simulink model "validation_gate_current"  (Simulink 7.6)
settings: Solver=FixedStepDiscrete  StartTime=0.0  StopTime=0  RelTol=1e-3
values from neighbouring files (symbols this model uses):
  Forward_Camera_Dimensions = [160 120]    [VisionConstants.m]
  Iter_Segment_Thresh = 60    [VisionConstants.m]
undefined symbols (not defined in the file or in its folder): Rec, SDTV
libraries: vipgeotforms x3, vipconversions x2, viptextngfix x1, vipanalysis x1, viptransforms x1
settings Model: Creator=Thing 1  LastModifiedBy=auvt
settings OptimizationCC: OptimizeModelRefInitCode=on
settings RTWCC: SystemTargetFile=ert.tlc  GenCodeOnly=on  TemplateMakefile=ert_default_tmf  Description=Real-Time Workshop Embedded Coder  GenerateReport=on  ProcessScript=ert_make_rtw_hook  IncludeHyperlinkInReport=on  LaunchReport=on  TargetLang=C++
settings CodeAppCC: IgnoreCustomStorageClasses=off
settings ERTTargetCC: MultiwordLength=2048  GenerateSampleERTMain=on  IncludeMdlTerminateFcn=off  ERTCustomFileTemplate=example_file_process.tlc  ConvertIfToSwitch=off

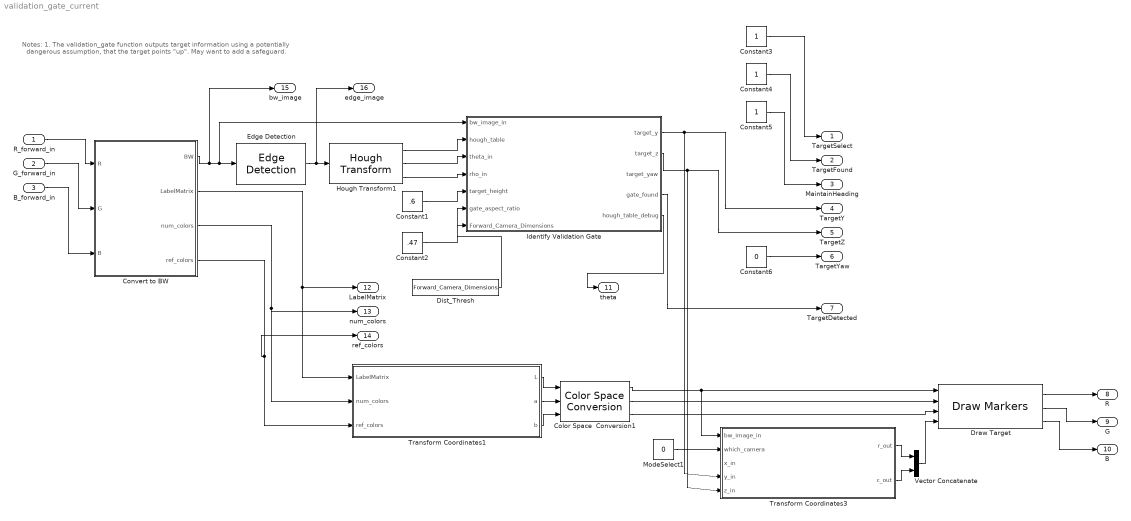
== system validation_gate_current ==
  note: Notes:
      | 1. The validation_gate function outputs target
      | information using a potentially dangerous
      | assumption, that the target points "up". May
      | want to add a safeguard.
  R_forward_in : Inport  PortDimensions=Forward_Camera_Dimensions
  G_forward_in : Inport  Port=2  PortDimensions=Forward_Camera_Dimensions
  B_forward_in : Inport  Port=3  PortDimensions=Forward_Camera_Dimensions
  Color Space  Conversion1 : vipconversions/Color Space  Conversion  conversion=Obsolete  conversionActive=L*a*b* to sR'G'B'  wp_str=D50  rec=Rec. 601 (SDTV)  sys=1125/60/2:1  imagePorts=Separate color signals
  Constant1 : Constant  Value=.6  SampleTime=-1
  Constant2 : Constant  Value=.47  SampleTime=-1
  Constant3 : Constant  SampleTime=-1
  Constant4 : Constant  SampleTime=-1
  Constant5 : Constant  SampleTime=-1
  Constant6 : Constant  Value=0  SampleTime=-1
  Convert to BW : Subsystem
  Dist_Thresh : Constant  Value=Forward_Camera_Dimensions  SampleTime=-1
  Draw Target : viptextngfix/Draw Markers  DialogController=vipDDGCreate  DialogControllerArgs=DataTag3  shape=X-mark  size=7  fill=off  fillClrSource=Specify via dialog  display=User-specified value  intensity=200  color=[0 0 0]  opacity=0.6  viewport=Entire image  antialiasing=off  inType=Obsolete  imagePorts=Separate color signals  prodOutputMode=Binary point scaling  prodOutputWordLength=32  prodOutputFracLength=14  memoryMode=Specify word length  memoryWordLength=16  memoryFracLength=15  roundingMode=Floor  overflowMode=off
  Edge Detection : vipanalysis/Edge Detection  DialogController=vipDDGCreate  DialogControllerArgs=DataTag4  method=Sobel  outputType=Binary image  userDefinedThreshold=off  thresholdSource=Specify via dialog  threshold=20  thresholdTuning=3  edgeThinning=on  threshold_canny=[0.25 0.60]  autoPercent=70  sigma=1  roundingMode=Floor  overflowMode=off
  Hough Transform1 : viptransforms/Hough Transform  DialogController=vipDDGCreate  DialogControllerArgs=DataTag5  theta_res=pi/180  rho_res=1  out_theta_rho=on  outdtmode=double  firstCoeffMode=Binary point scaling  firstCoeffWordLength=16  firstCoeffFracLength=14  secondCoeffMode=Binary point scaling  secondCoeffWordLength=32  secondCoeffFracLength=16  outputMode=Binary point scaling  outputWordLength=16  outputFracLength=0  accumMode=Binary point scaling  accumWordLength=32  accumFracLength=20  prodOutputMode=Binary point scaling  prodOutputWordLength=32  prodOutputFracLength=20  memoryMode=Binary point scaling  memoryWordLength=32  memoryFracLength=16  roundingMode=Nearest  overflowMode=on
  Identify Validation Gate : Stateflow chart  TreatAsAtomicUnit=on  SystemSampleTime=[1/30 0]
  ModeSelect1 : Constant  Value=0  SampleTime=-1
  Transform Coordinates1 : Stateflow chart  TreatAsAtomicUnit=on  SystemSampleTime=[1/30 0]
  Transform Coordinates3 : Stateflow chart  TreatAsAtomicUnit=on  SystemSampleTime=[1/30 0]
  Vector Concatenate : Concatenate  Mode=Multidimensional array
  TargetSelect : Outport  OutDataTypeStr=double
  TargetFound : Outport  Port=2  OutDataTypeStr=double
  MaintainHeading : Outport  Port=3  OutDataTypeStr=double
  TargetY : Outport  Port=4  OutDataTypeStr=double
  TargetZ : Outport  Port=5  OutDataTypeStr=double
  TargetYaw : Outport  Port=6  OutDataTypeStr=double
  TargetDetected : Outport  Port=7  OutDataTypeStr=double
  R : Outport  Port=8  OutDataTypeStr=double
  G : Outport  Port=9  OutDataTypeStr=double
  B : Outport  Port=10  OutDataTypeStr=double
  theta : Outport  Port=11  OutDataTypeStr=double
  LabelMatrix : Outport  Port=12
  num_colors : Outport  Port=13
  ref_colors : Outport  Port=14
  bw_image : Outport  Port=15
  edge_image : Outport  Port=16
  wires:
  Hough Transform1/1 -> Identify Validation Gate/2(hough_table)
  Hough Transform1/2 -> Identify Validation Gate/3(theta_in)
  Hough Transform1/3 -> Identify Validation Gate/4(rho_in)
  Edge Detection/1 -> Hough Transform1/1, edge_image/1
  Constant1/1 -> Identify Validation Gate/5(target_height)
  Constant2/1 -> Identify Validation Gate/6(gate_aspect_ratio)
  Convert to BW/1(BW) -> Edge Detection/1, Identify Validation Gate/1(bw_image_in), bw_image/1
  R_forward_in/1 -> Convert to BW/1(R)
  G_forward_in/1 -> Convert to BW/2(G)
  B_forward_in/1 -> Convert to BW/3(B)
  Identify Validation Gate/1(target_y) -> TargetY/1, Transform Coordinates3/4(y_in)
  Identify Validation Gate/2(target_z) -> TargetZ/1, Transform Coordinates3/5(z_in)
  Identify Validation Gate/4(gate_found) -> TargetDetected/1
  Constant3/1 -> TargetSelect/1
  Constant4/1 -> TargetFound/1
  Constant5/1 -> MaintainHeading/1
  Constant6/1 -> TargetYaw/1
  Vector Concatenate/1 -> Draw Target/4
  Transform Coordinates3/1(r_out) -> Vector Concatenate/1
  Transform Coordinates3/2(c_out) -> Vector Concatenate/2
  ModeSelect1/1 -> Transform Coordinates3/2(which_camera)
  Draw Target/1 -> R/1
  Draw Target/2 -> G/1
  Draw Target/3 -> B/1
  Transform Coordinates1/1(L) -> Color Space  Conversion1/1
  Transform Coordinates1/2(a) -> Color Space  Conversion1/2
  Transform Coordinates1/3(b) -> Color Space  Conversion1/3
  Color Space  Conversion1/1 -> Draw Target/1, Transform Coordinates3/1(bw_image_in)
  Color Space  Conversion1/2 -> Draw Target/2
  Color Space  Conversion1/3 -> Draw Target/3
  Convert to BW/2(LabelMatrix) -> Transform Coordinates1/1(LabelMatrix), LabelMatrix/1
  Convert to BW/3(num_colors) -> Transform Coordinates1/2(num_colors), num_colors/1
  Convert to BW/4(ref_colors) -> Transform Coordinates1/3(ref_colors), ref_colors/1
  Identify Validation Gate/5(hough_table_debug) -> theta/1
  Dist_Thresh/1 -> Identify Validation Gate/7(Forward_Camera_Dimensions)

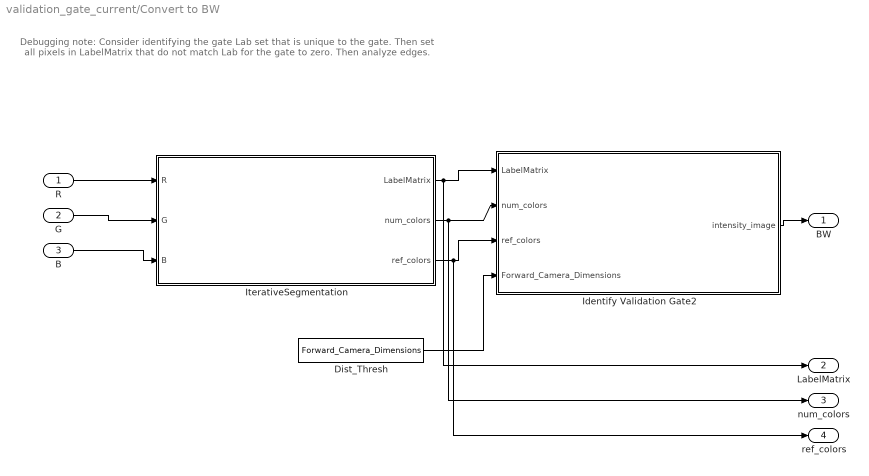
== system validation_gate_current/Convert to BW ==
  note: Debugging note: Consider identifying the gate Lab set that is unique to the gate.
      | Then set all pixels in LabelMatrix that do not match Lab for the gate to zero.
      | Then analyze edges.
  R : Inport  OutDataTypeStr=double
  G : Inport  Port=2  OutDataTypeStr=double
  B : Inport  Port=3  OutDataTypeStr=double
  Dist_Thresh : Constant  Value=Forward_Camera_Dimensions  SampleTime=-1
  Identify Validation Gate2 : Stateflow chart  TreatAsAtomicUnit=on  SystemSampleTime=[1/30 0]
  IterativeSegmentation : Subsystem
      settings: UndoDeleteFcn=Stateflow.SLINSF.SimulinkMan.restorePreDeleteFcn  PreDeleteFcn=Stateflow.SLINSF.SimulinkMan.removePreDeleteFcn
  BW : Outport
  LabelMatrix : Outport  Port=2
  num_colors : Outport  Port=3
  ref_colors : Outport  Port=4
  wires:
  R/1 -> IterativeSegmentation/1(R)
  G/1 -> IterativeSegmentation/2(G)
  B/1 -> IterativeSegmentation/3(B)
  Identify Validation Gate2/1(intensity_image) -> BW/1
  IterativeSegmentation/1(LabelMatrix) -> Identify Validation Gate2/1(LabelMatrix), LabelMatrix/1
  IterativeSegmentation/2(num_colors) -> Identify Validation Gate2/2(num_colors), num_colors/1
  IterativeSegmentation/3(ref_colors) -> Identify Validation Gate2/3(ref_colors), ref_colors/1
  Dist_Thresh/1 -> Identify Validation Gate2/4(Forward_Camera_Dimensions)

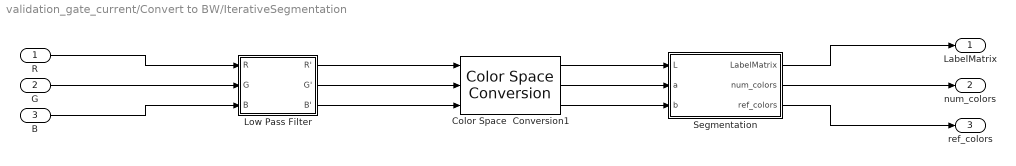
== system validation_gate_current/Convert to BW/IterativeSegmentation ==
  R : Inport
  G : Inport  Port=2
  B : Inport  Port=3
  Color Space  Conversion1 : vipconversions/Color Space  Conversion  conversion=Obsolete  conversionActive=sR'G'B' to L*a*b*  wp_str=D50  rec=Rec. 601 (SDTV)  sys=1125/60/2:1  imagePorts=Separate color signals
  Low Pass Filter : Subsystem
  Segmentation : Subsystem
  LabelMatrix : Outport
  num_colors : Outport  Port=2
  ref_colors : Outport  Port=3
  wires:
  Segmentation/3(ref_colors) -> ref_colors/1
  Segmentation/2(num_colors) -> num_colors/1
  Segmentation/1(LabelMatrix) -> LabelMatrix/1
  Low Pass Filter/3(B') -> Color Space  Conversion1/3
  Low Pass Filter/2(G') -> Color Space  Conversion1/2
  Low Pass Filter/1(R') -> Color Space  Conversion1/1
  Color Space  Conversion1/3 -> Segmentation/3(b)
  Color Space  Conversion1/2 -> Segmentation/2(a)
  Color Space  Conversion1/1 -> Segmentation/1(L)
  R/1 -> Low Pass Filter/1(R)
  G/1 -> Low Pass Filter/2(G)
  B/1 -> Low Pass Filter/3(B)

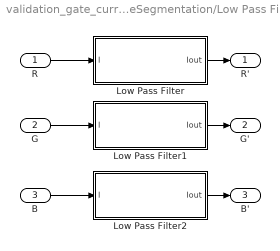
== system validation_gate_current/Convert to BW/IterativeSegmentation/Low Pass Filter ==
  R : Inport
  G : Inport  Port=2
  B : Inport  Port=3
  Low Pass Filter : Stateflow chart  TreatAsAtomicUnit=on
  Low Pass Filter1 : Stateflow chart  TreatAsAtomicUnit=on
  Low Pass Filter2 : Stateflow chart  TreatAsAtomicUnit=on
  R' : Outport
  G' : Outport  Port=2
  B' : Outport  Port=3
  wires:
  Low Pass Filter/1(Iout) -> R'/1
  Low Pass Filter2/1(Iout) -> B'/1
  Low Pass Filter1/1(Iout) -> G'/1
  B/1 -> Low Pass Filter2/1(I)
  G/1 -> Low Pass Filter1/1(I)
  R/1 -> Low Pass Filter/1(I)

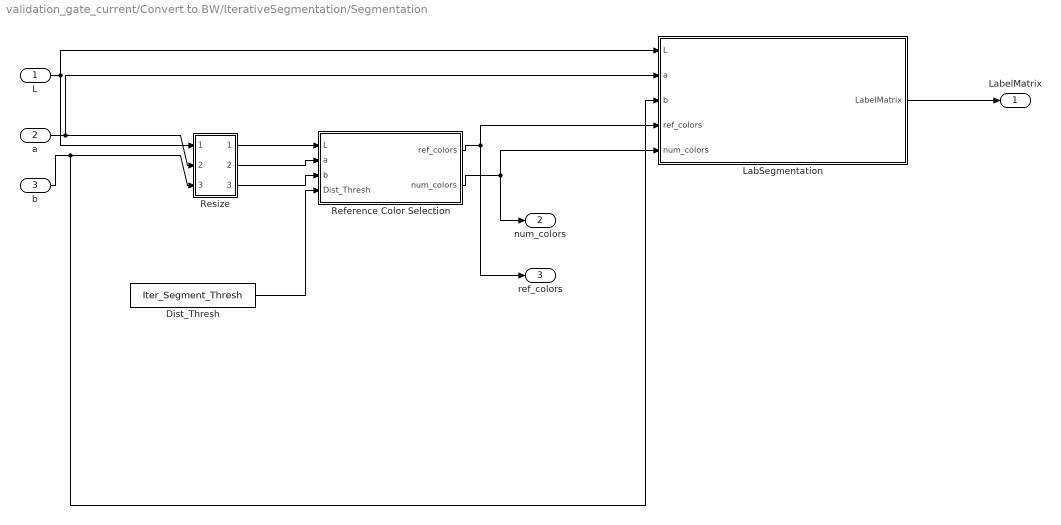
== system validation_gate_current/Convert to BW/IterativeSegmentation/Segmentation ==
  L : Inport
  a : Inport  Port=2
  b : Inport  Port=3
  Dist_Thresh : Constant  Value=Iter_Segment_Thresh  SampleTime=-1
  LabSegmentation : Stateflow chart  TreatAsAtomicUnit=on
  Reference Color Selection : Stateflow chart  TreatAsAtomicUnit=on
  Resize : Subsystem
  LabelMatrix : Outport
  num_colors : Outport  Port=2
  ref_colors : Outport  Port=3
  wires:
  Dist_Thresh/1 -> Reference Color Selection/4(Dist_Thresh)
  LabSegmentation/1(LabelMatrix) -> LabelMatrix/1
  Reference Color Selection/2(num_colors) -> LabSegmentation/5(num_colors), num_colors/1
  Reference Color Selection/1(ref_colors) -> ref_colors/1, LabSegmentation/4(ref_colors)
  Resize/3(Out3) -> Reference Color Selection/3(b)
  Resize/2(Out2) -> Reference Color Selection/2(a)
  Resize/1(Out1) -> Reference Color Selection/1(L)
  b/1 -> LabSegmentation/3(b), Resize/3(In3)
  a/1 -> LabSegmentation/2(a), Resize/2(In2)
  L/1 -> LabSegmentation/1(L), Resize/1(In1)

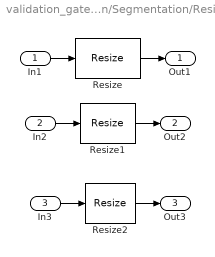
== system validation_gate_current/Convert to BW/IterativeSegmentation/Segmentation/Resize ==
  In1 : Inport
  In2 : Inport  Port=2
  In3 : Inport  Port=3
  Resize : vipgeotforms/Resize  DialogController=vipDDGCreate  DialogControllerArgs=DataTag0  specify=Number of output rows and columns  rfactor=[]  outCols=25  outRows=25  outRowsCols=[60 80]  interp_method=Bilinear  antialias=on  useROI=off  roiFlag=off  prodOutputMode=Binary point scaling  prodOutputWordLength=32  prodOutputFracLength=10  roundingMode=Nearest  overflowMode=on
  Resize1 : vipgeotforms/Resize  DialogController=vipDDGCreate  DialogControllerArgs=DataTag1  specify=Number of output rows and columns  rfactor=[200 150]  outCols=25  outRows=25  outRowsCols=[60 80]  interp_method=Bilinear  antialias=on  useROI=off  roiFlag=off  prodOutputMode=Binary point scaling  prodOutputWordLength=32  prodOutputFracLength=10  roundingMode=Nearest  overflowMode=on
  Resize2 : vipgeotforms/Resize  DialogController=vipDDGCreate  DialogControllerArgs=DataTag2  specify=Number of output rows and columns  rfactor=[200 150]  outCols=25  outRows=25  outRowsCols=[60 80]  interp_method=Bilinear  antialias=on  useROI=off  roiFlag=off  prodOutputMode=Binary point scaling  prodOutputWordLength=32  prodOutputFracLength=10  roundingMode=Nearest  overflowMode=on
  Out1 : Outport
  Out2 : Outport  Port=2
  Out3 : Outport  Port=3
  wires:
  Resize2/1 -> Out3/1
  In3/1 -> Resize2/1
  Resize1/1 -> Out2/1
  In2/1 -> Resize1/1
  Resize/1 -> Out1/1
  In1/1 -> Resize/1

== matlab function Identify Validation Gate ==
  data: bw_image_in input double; hough_table input double; target_y output double; target_z output double; target_yaw output double; gate_found output double; theta_in input double; rho_in input double; target_height input double; gate_aspect_ratio input double; hough_table_debug output double; Forward_Camera_Dimensions input double
function [target_y, target_z, target_yaw, gate_found, hough_table_debug] = validation_gate(bw_image_in, hough_table, theta_in, rho_in, target_height, gate_aspect_ratio, Forward_Camera_Dimensions)
%#eml



% This function attempts to identfiy the validation gate, and returns
%   targeting information, and a true/false gate_found parameter.
%
% 5-29-11
%
% Input
%
%   target_height = fraction of goal post height to aim AUV at
%   gate_aspect_ratio = used to infer unknown points with little extra
%     processing (height/width of large goalpost-shape)
%
% Output
%
% Notes:
%   The hough_table is destroyed in this function (acceptable if
%     hough_table is not an output)
%   Process:
%     1. Identify primary, relatively "long" lines
%     2. 


%% Initialize
% Only the (max_num_lines) with the most votes will be considered as
%   candidates for the validation gate
max_num_lines = 200;
[rho_length, theta_length] = size(hough_table);
%[rows, cols] = size(bw_image_in);
%rows = Forward_Camera_Dimensions(1);
%cols = Forward_Camera_Dimensions(2);
rows = 160;
cols = 120;



% eps_rho must be at least as big as the gate leg diameter (units of
%   pixels)
eps_rho = .1*max(rows,cols);
% eps_theta is used to distinguish lines as "horizontal" or "vertical";
%   units are radians
eps_theta = 10*pi/180;


% These vectors contain the final three lines that compose the validation gate
rho_gate = zeros(1,3);
theta_gate = zeros(1,3);

% These vectors contain intermediate line information; as lines are
%   eliminated from these vectors, their values are set to zero
rho = zeros(1,max_num_lines);
theta = zeros(1,max_num_lines);





% Identify the most popular max_num_lines lines
i_index = ones(1,max_num_lines);
j_index = ones(1,max_num_lines);

m = 1;
while( m <= max_num_lines )
    
    max_votes = 0;
    for i = 1:rho_length
        for j = 1:theta_length
            if( hough_table(i,j) > max_votes )
                i_index(m) = i;
                j_index(m) = j;
                max_votes = hough_table(i,j);
            end
        end
    end
    
    rho(m) = rho_in(i_index(m));
    theta(m) = theta_in(j_index(m));
    hough_table(i_index(m),j_index(m)) = 0;
    m = m + 1;
    
end


% Effectively generate a small Hough table which contains only values of
%   interest for the validation gate application

rbinv = [0:(2*eps_rho):max(rows, cols)];  % Rho bins for vertical lines
nbinsv = length(rbinv);  % Number of rho bins for vertical lines
ravgv = zeros(1,nbinsv);  % Average rho values for each bin (note that the average value will generally differ slightly than the bin value)
tavgv = zeros(1,nbinsv);  % Average theta values for each bin
vbinv = zeros(1,nbinsv);  % Votes bins for vertical lines

rbinh = [0:(2*eps_rho):max(rows, cols)];
nbinsh = length(rbinh);
ravgh = zeros(1,nbinsh);
tavgh = zeros(1,nbinsh);
vbinh = zeros(1,nbinsh);

% Allow vertical lines along the left side of the image
rbinv(1) = 1;
rbinh(1) = 1;

for i = 1:max_num_lines
    
    % Consider only lines that are either vertical or horizontal, within
    %   tolerance
    condition1 = ( abs(theta(i) - pi/2) <= eps_theta || abs(theta(i) + pi/2) <= eps_theta );  % Horizontal line
    condition2 = ( abs(theta(i) - 0) <= eps_theta );  % Vertical line
    
    if(condition2 && ~( rho(i) == 0 && theta(i) == 0 ))  % Analyze vertical lines (ignore lines exactly along the left side of the image)
        
        for b = 1:nbinsv
            
            % Place each rho value into a bin
            if( abs(rho(i) - rbinv(b)) <= eps_rho )
                ravgv(b) = ravgv(b) + rho(i);
                tavgv(b) = tavgv(b) + theta(i);
                vbinv(b) = vbinv(b) + 1;
                break;
            end
            
        end
        
    elseif(condition1)  % Analyze horizontal lines
        
        if( theta(i) < 0 )
            theta(i) = theta(i) + pi;
            rho(i) = -rho(i);
        end
        
        for b = 1:nbinsh
            
            % Place each rho value into a bin
            if( abs(rho(i) - rbinh(b)) <= eps_rho )
                ravgh(b) = ravgh(b) + rho(i);
                tavgh(b) = tavgh(b) + theta(i);
                vbinh(b) = vbinh(b) + 1;
                break;
            end
            
        end
        
    end
end

% Average the values in ravg and tavg for horizontal and vertical lines
for b = 1:nbinsv
    if( vbinv(b) == 0 )
        ravgv(b) = 0;
        tavgv(b) = 0;
    else
        ravgv(b) = ravgv(b)./vbinv(b);
        tavgv(b) = tavgv(b)./vbinv(b);
    end
end
for b = 1:nbinsh
    if( vbinh(b) == 0 )
        ravgh(b) = 0;
        tavgh(b) = 0;
    else
        ravgh(b) = ravgh(b)./vbinh(b);
        tavgh(b) = tavgh(b)./vbinh(b);
    end
end


%% Extract three lines that fit the criteria for being the validation gate
rmin = 10000;
rmax = -10000;
for b = 1:nbinsv
    
    % Extract the left-most vertical line
    if( ravgv(b) < rmin && ravgv(b) ~= 0 )
        rmin = ravgv(b);
        rho_gate(1) = ravgv(b);
        theta_gate(1) = tavgv(b);
    end
    
    % Extract the right-most vertical line
    if( ravgv(b) > rmax && ravgv(b) ~= 0 )
        rmax = ravgv(b);
        rho_gate(3) = ravgv(b);
        theta_gate(3) = tavgv(b);
    end
    
end

% Check that the distance between the vertical lines is much greater than
%   the minimum expected distance, eps_rho
if( abs(rho_gate(3) - rho_gate(1)) < 2*eps_rho )
    rho_gate(1) = 0;
    rho_gate(3) = 0;
    theta_gate(1) = 0;
    theta_gate(3) = 0;
end

%rmin = 10000;
vmax = 0;
for b = 1:nbinsh
    
    % Extract the horizontal line with the most votes
    if( vbinh(b) > vmax && ravgh(b) ~= 0 )
        vmax = vbinh(b);
        rho_gate(2) = ravgh(b);
        theta_gate(2) = tavgh(b);
    end
    
%    % Extract the horizontal line that is highest up in the image
%    if( ravgh(b) < rmin && ravgh(b) ~= 0 )
%        rmin = ravgh(b);
%        rho_gate(2) = ravgh(b);
%        theta_gate(2) = tavgh(b);
%    end
end


%% Compute targeting information
% Compute intersections
r1 = (  ( rho_gate(1)/cos(theta_gate(1)) ) - ( rho_gate(2)/cos(theta_gate(2)) )  )*(  1/( tan(theta_gate(1)) - tan(theta_gate(2)) )  );
c1 = ( 1/cos(theta_gate(1)) )*( rho_gate(1) - r1*sin(theta_gate(1)) );

r3 = (  ( rho_gate(2)/cos(theta_gate(2)) ) - ( rho_gate(3)/cos(theta_gate(3)) )  )*(  1/( tan(theta_gate(2)) - tan(theta_gate(3)) )  );
c3 = ( 1/cos(theta_gate(2)) )*( rho_gate(2) - r3*sin(theta_gate(2)) );

r2 = (r1 + r3)/2;
c2 = (c1 + c3)/2;

% Compute gate width
w = sqrt( (r3 - r1)^2 + (c3 - c1)^2 );

% Form unit vector pointing downward, parallel to gate posts
tavg = ( theta_gate(1) + (theta_gate(2) - pi/2) + theta_gate(3) )/3;
u = [1 tan(tavg)];
u = u./norm(u);

% Compute target location
th = target_height*gate_aspect_ratio*w;
r_t = r2 + th*u(1);
c_t = c2 + th*u(2);

% Determine if a gate is present (very simple, potentially inaccurate)
if( sum( (rho_gate == 0) + (theta_gate == 0) ) > 0 )
    
    gate_found = 0;
    target_z = 0;
    target_y = 0;
    
else
    
    gate_found = 1;
    
    % Transform target r, c to global coordinate system
    target_z = r_t - floor(rows/2);
    target_y = c_t - floor(cols/2);
    
end

target_y = 180*theta(1)/pi;
target_z = 180*theta(2)/pi;
target_yaw = pi;

hough_table_debug = hough_table;

return

== matlab function Transform Coordinates3 ==
  data: bw_image_in input double; which_camera input double; x_in input double; y_in input double; r_out output double; c_out output double; z_in input double
function [r_out, c_out] = transform_G2L(bw_image_in, which_camera, x_in, y_in, z_in)
% This function, "transform Global to Local coordinates," transforms
%   global coordinates that are sent to the controller into local
%   coordinates that can be displayed over images.
%
% 5-29-11
%
% Input
%   x_in, y_in, z_in = vectors of points in global (vehicle-centered)
%     coordinate system
%   bw_image_in = a 2-D array of pixel values (used only to extract image
%     size)
%   which_camera = selects which camera for relative coordinates
%                = 0 -> Forward camera
%                = 1 -> Down camera
%
% Output
%   r_out, c_out = row, column pairs in local coordinate system

[rows, cols] = size(bw_image_in);
if( which_camera == 0 )
    r_out = z_in + floor(rows/2);
    c_out = y_in + floor(cols/2);
else
    r_out = floor(rows/2) - x_in;
    c_out = y_in + floor(cols/2);
end

%{
if( which_camera == 0 )
    r_out = int32( z_in + floor(rows/2) );
    c_out = int32( y_in + floor(cols/2) );
else
    r_out = int32( floor(rows/2) - x_in );
    c_out = int32( y_in + floor(cols/2) );
end
%}
return

== matlab function Convert to BW/Identify Validation Gate2 ==
  data: LabelMatrix input double; intensity_image output double; num_colors input double; ref_colors input double; Forward_Camera_Dimensions input double
function intensity_image  = makeIntensityImage(LabelMatrix, num_colors, ref_colors, Forward_Camera_Dimensions)
%#eml


% Initialize
max_num_cols = 2;
%[rows, cols] = size(LabelMatrix);
%rows = Forward_Camera_Dimensions(1);
%cols = Forward_Camera_Dimensions(2);

rows = 160;
cols = 120;
intensity_image = zeros(rows, cols);
%intensity_image = zeros(160 120);


maxL = zeros(1, max_num_cols);
gate_i = ones(1, max_num_cols);


% Identify max_num_cols colors with the brightest L color components
for n = 1:max_num_cols
    
    for i = 1:num_colors
        if( ref_colors(i,1) > maxL(n) )
            gate_i(n) = i;
            maxL(n) = ref_colors(i,1);
        end
    end
    
    ref_colors(gate_i(n),1) = -1;
    
end


% Ignore all non-white values
for r = 1:rows
    for c = 1:cols
        
        for n = 1:max_num_cols
            if( LabelMatrix(r,c) == gate_i(n) )
                intensity_image(r,c) = 1;
            end
        end
        
    end
end


return

== matlab function Transform Coordinates1 ==
  data: LabelMatrix input double; num_colors input double; ref_colors input double; L output double; a output double; b output double
function [L, a, b] = displaySegmentedImage(LabelMatrix, num_colors, ref_colors)


intensity_image = LabelMatrix./max(max(max(abs(LabelMatrix))));


[rows, cols] = size(LabelMatrix);

L = zeros(rows, cols);
a = zeros(rows, cols);
b = zeros(rows, cols);

for r = 1:rows
    for c = 1:cols
        L(r,c) = ref_colors(LabelMatrix(r,c), 1);
        a(r,c) = ref_colors(LabelMatrix(r,c), 2);
        b(r,c) = ref_colors(LabelMatrix(r,c), 3);
    end
end

return

== matlab function Convert to BW/IterativeSegmentation/Low Pass Filter/Low Pass Filter ==
  data: I input double; Iout output double
function Iout = GaussianBlurr(I)
% This function calculates the gaussian blur of an intensity image

sigma = sqrt(2);

Grows = 3;    % Gaussian matrix rows
Gcols = 3;    % Gaussian matrix columns

[Irows Icols] = size(I);

Iout = double(zeros(Irows,Icols));

Trows = Irows - Grows + 1;
Tcols = Icols - Gcols + 1;
Itemp = double(zeros(Trows,Tcols));

G = zeros(Grows,Gcols);

FirstRow = ceil(-Grows/2);
LastRow = floor(Grows/2);
FirstCol = ceil(-Gcols/2);
LastCol = floor(Gcols/2);
Gsum = 0;
for i=FirstRow:LastRow
    for j = FirstCol:LastCol
        G(i-FirstRow+1,j-FirstCol+1) = exp(-(j*j+i*i)/(2*sigma*sigma));
        Gsum = Gsum + G(i-FirstRow+1,j-FirstCol+1);
    end
end

G = G./Gsum;

Itemp = conv2(double(I),double(G),'valid');

% reflect boundaries to keep image the same size
% top
Iout((1:LastRow),(LastCol+1:Icols-LastCol)) = Itemp((1:LastRow),(1:Tcols));
% bottom
Iout((Irows-LastRow+1:Irows),(LastCol+1:Icols-LastCol)) = Itemp((Trows-LastRow+1:Trows),(1:Tcols));
% left
Iout((1+LastRow:Irows-LastRow),(1:LastCol)) = Itemp((1:Trows),(1:LastCol));
% right
Iout((1+LastRow:Irows-LastRow),(Icols-LastCol+1:Icols)) = Itemp((1:Trows),(Tcols-LastCol+1:Tcols));
% center
Iout((1+LastRow:Irows-LastRow),(1+LastCol:Icols-LastCol)) = Itemp;
% top left corner
Iout(1:LastRow,1:LastCol) = Itemp(1:LastRow,1:LastCol);
% top right corner
Iout(1:LastRow,Icols-LastCol:Icols) = Itemp(1:LastRow,Tcols-LastCol:Tcols);
% bottom left corner
Iout(Irows-LastRow:Irows,1:LastCol) = Itemp(Trows-LastRow:Trows,1:LastCol);
% bottom right corner
Iout(Irows-LastRow:Irows,Icols-LastCol:Icols) = Itemp(Trows-LastRow:Trows,Tcols-LastCol:Tcols);

return

== matlab function Convert to BW/IterativeSegmentation/Low Pass Filter/Low Pass Filter1 ==
  data: I input double; Iout output double
function Iout = GaussianBlurr(I)
% This function calculates the gaussian blur of an intensity image

sigma = sqrt(2);

Grows = 3;    % Gaussian matrix rows
Gcols = 3;    % Gaussian matrix columns

[Irows Icols] = size(I);

Iout = double(zeros(Irows,Icols));

Trows = Irows - Grows + 1;
Tcols = Icols - Gcols + 1;
Itemp = double(zeros(Trows,Tcols));

G = zeros(Grows,Gcols);

FirstRow = ceil(-Grows/2);
LastRow = floor(Grows/2);
FirstCol = ceil(-Gcols/2);
LastCol = floor(Gcols/2);
Gsum = 0;
for i=FirstRow:LastRow
    for j = FirstCol:LastCol
        G(i-FirstRow+1,j-FirstCol+1) = exp(-(j*j+i*i)/(2*sigma*sigma));
        Gsum = Gsum + G(i-FirstRow+1,j-FirstCol+1);
    end
end

G = G./Gsum;

Itemp = conv2(double(I),double(G),'valid');

% reflect boundaries to keep image the same size
% top
Iout((1:LastRow),(LastCol+1:Icols-LastCol)) = Itemp((1:LastRow),(1:Tcols));
% bottom
Iout((Irows-LastRow+1:Irows),(LastCol+1:Icols-LastCol)) = Itemp((Trows-LastRow+1:Trows),(1:Tcols));
% left
Iout((1+LastRow:Irows-LastRow),(1:LastCol)) = Itemp((1:Trows),(1:LastCol));
% right
Iout((1+LastRow:Irows-LastRow),(Icols-LastCol+1:Icols)) = Itemp((1:Trows),(Tcols-LastCol+1:Tcols));
% center
Iout((1+LastRow:Irows-LastRow),(1+LastCol:Icols-LastCol)) = Itemp;
% top left corner
Iout(1:LastRow,1:LastCol) = Itemp(1:LastRow,1:LastCol);
% top right corner
Iout(1:LastRow,Icols-LastCol:Icols) = Itemp(1:LastRow,Tcols-LastCol:Tcols);
% bottom left corner
Iout(Irows-LastRow:Irows,1:LastCol) = Itemp(Trows-LastRow:Trows,1:LastCol);
% bottom right corner
Iout(Irows-LastRow:Irows,Icols-LastCol:Icols) = Itemp(Trows-LastRow:Trows,Tcols-LastCol:Tcols);

return

== matlab function Convert to BW/IterativeSegmentation/Low Pass Filter/Low Pass Filter2 ==
  data: I input double; Iout output double
function Iout = GaussianBlurr(I)
% This function calculates the gaussian blur of an intensity image

sigma = sqrt(2);

Grows = 3;    % Gaussian matrix rows
Gcols = 3;    % Gaussian matrix columns

[Irows Icols] = size(I);

Iout = double(zeros(Irows,Icols));

Trows = Irows - Grows + 1;
Tcols = Icols - Gcols + 1;
Itemp = double(zeros(Trows,Tcols));

G = zeros(Grows,Gcols);

FirstRow = ceil(-Grows/2);
LastRow = floor(Grows/2);
FirstCol = ceil(-Gcols/2);
LastCol = floor(Gcols/2);
Gsum = 0;
for i=FirstRow:LastRow
    for j = FirstCol:LastCol
        G(i-FirstRow+1,j-FirstCol+1) = exp(-(j*j+i*i)/(2*sigma*sigma));
        Gsum = Gsum + G(i-FirstRow+1,j-FirstCol+1);
    end
end

G = G./Gsum;

Itemp = conv2(double(I),double(G),'valid');

% reflect boundaries to keep image the same size
% top
Iout((1:LastRow),(LastCol+1:Icols-LastCol)) = Itemp((1:LastRow),(1:Tcols));
% bottom
Iout((Irows-LastRow+1:Irows),(LastCol+1:Icols-LastCol)) = Itemp((Trows-LastRow+1:Trows),(1:Tcols));
% left
Iout((1+LastRow:Irows-LastRow),(1:LastCol)) = Itemp((1:Trows),(1:LastCol));
% right
Iout((1+LastRow:Irows-LastRow),(Icols-LastCol+1:Icols)) = Itemp((1:Trows),(Tcols-LastCol+1:Tcols));
% center
Iout((1+LastRow:Irows-LastRow),(1+LastCol:Icols-LastCol)) = Itemp;
% top left corner
Iout(1:LastRow,1:LastCol) = Itemp(1:LastRow,1:LastCol);
% top right corner
Iout(1:LastRow,Icols-LastCol:Icols) = Itemp(1:LastRow,Tcols-LastCol:Tcols);
% bottom left corner
Iout(Irows-LastRow:Irows,1:LastCol) = Itemp(Trows-LastRow:Trows,1:LastCol);
% bottom right corner
Iout(Irows-LastRow:Irows,Icols-LastCol:Icols) = Itemp(Trows-LastRow:Trows,Tcols-LastCol:Tcols);

return

== matlab function Convert to BW/IterativeSegmentation/Segmentation/LabSegmentation ==
  data: L input double; LabelMatrix output double; a input double; b input double; ref_colors input double; num_colors input double
function LabelMatrix  = LabSegmentation(L,a,b,ref_colors,num_colors)
% This function generates the label matrix

[rows cols] = size(L);

Lout = zeros(rows,cols);
aout = zeros(rows,cols);
bout = zeros(rows,cols);

LabelMatrix = zeros(rows,cols);

for i = 1:rows
    for j = 1:cols
        min_dist = 1000;
        index = 1;
        for k = 1:num_colors
            dist = sqrt((ref_colors(k,1) - L(i,j))^2 + (ref_colors(k,2) - a(i,j))^2 + (ref_colors(k,3) - b(i,j))^2);
            if(dist < min_dist)
                min_dist = double(dist);
                index = k;
            end
        end
        LabelMatrix(i,j) = index;
    end
end

for i = 1:rows
    for j = 1:cols
        Lout(i,j) = ref_colors(LabelMatrix(i,j),1);
        aout(i,j) = ref_colors(LabelMatrix(i,j),2);
        bout(i,j) = ref_colors(LabelMatrix(i,j),3);
    end
end

cow = 1;

return

== matlab function Convert to BW/IterativeSegmentation/Segmentation/Reference Color Selection ==
  data: L input double; ref_colors output double; a input double; b input double; num_colors output double; Dist_Thresh input double
function [ref_colors, num_colors] = Segmentation(L,a,b,Dist_Thresh)
% This function tries segmentation by adding new reference colors everytime
% a pixel is found with a distance greater than a certain amount from
% every other reference color

[rows cols] = size(L);

Dist_Threshold = Dist_Thresh;% L = 0 to 100, a = -100 to 100, b = -100 to 100
                    % max dist = 300 -> 60/300 is 20%
x = 1;  % coefficients determining distance calculation
y = 1.5;
z = 1.5;

max_num_colors = 50;
ref_colors = zeros(max_num_colors,3);   % At most 50 different reference colors
LabelMatrix = zeros(rows,cols);
num_colors = 1;

center_row = floor(rows/2);
center_col = floor(cols/2);

% Define first reference color to be colr
ref_colors(1,:) = [L(center_row,center_col) a(center_row,center_col) b(center_row,center_col)];

flag = 0;
i = 1;
j = 1;
while(i <= rows)        % perform initial segmentation
    while(i <= rows && flag == 0)
        while(j <= cols && flag == 0)
            k = 1;
            min_dist = 1000;
            index = 1;
            while(k <= num_colors)
                dist = sqrt(x*(ref_colors(k,1) - L(i,j))^2 + y*(ref_colors(k,2) - a(i,j))^2 + z*(ref_colors(k,3) - b(i,j))^2);
                if(min_dist > dist)
                    min_dist = double(dist);
                    index = k;
                end
                k = k + 1;
            end
            if(j == 117)
                cow = 1;
            end
            if(min_dist > Dist_Threshold && num_colors < max_num_colors)
                ref_colors(num_colors+1,:) = [L(i,j) a(i,j) b(i,j)];
                num_colors = num_colors + 1;
                flag = 1;
                i = 0;
                j = 0;
            else
                LabelMatrix(i,j) = index;
            end
            j = j + 1;
        end
        j = 1;
        i = i + 1;
    end
    flag = 0;
end

% Go through image once more to get more accurate values for the different regions
ref_color_L_avg = zeros(50,1);
ref_color_a_avg = zeros(50,1);
ref_color_b_avg = zeros(50,1);
color_count = zeros(50,1);
for i = 1:rows
    for j = 1:cols
        index = LabelMatrix(i,j);
        ref_color_L_avg(index) = ref_color_L_avg(index) + L(i,j);
        ref_color_a_avg(index) = ref_color_a_avg(index) + a(i,j);
        ref_color_b_avg(index) = ref_color_b_avg(index) + b(i,j);
        color_count(index) = color_count(index) + 1;
    end
end
ref_color_L_avg = ref_color_L_avg ./ color_count;
ref_color_a_avg = ref_color_a_avg ./ color_count;
ref_color_b_avg = ref_color_b_avg ./ color_count;

for i = 1:num_colors
    ref_colors(i,1) = ref_color_L_avg(i);
    ref_colors(i,2) = ref_color_a_avg(i);
    ref_colors(i,3) = ref_color_b_avg(i);
end

return
